simulink model "crazyflie_simulation_paper"  (R2019a)
settings: Solver=FixedStepAuto  StartTime=0.0  StopTime=50  FixedStep=Ts  RelTol=1e-3
values from neighbouring files (symbols this model uses):
  b = 0.033    [CHANGE_set_params_paper.m]    (also in set_params.m; set_params_paper.m)
  D_0 = 4/(Ts^2) + 4*zeta*omega_n/Ts + omega_n^2    (= 1011376)    [CHANGE_set_params_paper.m]    (also in set_params.m = 1057500; set_params_paper.m = 1057500)
  D_1 = -8/(Ts^2) + 2*omega_n^2    (= -1999872)    [CHANGE_set_params_paper.m]    (also in set_params.m = -1995000; set_params_paper.m = -1995000)
  D_2 = 4/(Ts^2) - 4*zeta*omega_n/Ts + omega_n^2    (= 988752)    [CHANGE_set_params_paper.m]    (also in set_params.m = 947500; set_params_paper.m = 947500)
  g = 9.81    [CHANGE_set_params_paper.m]    (also in set_params.m; set_params_paper.m)
  I_CF_1 = [16.823890  -1.224320  -0.716891 ... (first row only)    [CHANGE_set_params_paper.m]    (also in set_params.m; set_params_paper.m)
  I_CF_1_inv = inv(I_CF_1)    [CHANGE_set_params_paper.m]    (also in set_params.m; set_params_paper.m)
  I_rzz = 9.3e-9    (= 9.3e-09)    [CHANGE_set_params_paper.m]    (also in set_params.m; set_params_paper.m)
  k_f = 1.6e-4    (= 0.00016)    [CHANGE_set_params_paper.m]    (also in set_params.m; set_params_paper.m)
  k_m = 1e-6    (= 1e-06)    [CHANGE_set_params_paper.m]    (also in set_params.m; set_params_paper.m)
  kx = 10.25e-4    (= 0.001025)    [CHANGE_set_params_paper.m]    (also in set_params.m; set_params_paper.m)
  ky = 10.25e-4    (= 0.001025)    [CHANGE_set_params_paper.m]    (also in set_params.m; set_params_paper.m)
  kz = 7.553e-4    (= 0.0007553)    [CHANGE_set_params_paper.m]    (also in set_params.m; set_params_paper.m)
  l = 0.033    [CHANGE_set_params_paper.m]    (also in set_params.m; set_params_paper.m)
  m_CF = 0.028    [CHANGE_set_params_paper.m]    (also in set_params.m; set_params_paper.m)
  N_0 = omega_n^2    (= 64)    [CHANGE_set_params_paper.m]    (also in set_params.m = 2500; set_params_paper.m = 2500)
  N_1 = 2*omega_n^2    (= 128)    [CHANGE_set_params_paper.m]    (also in set_params.m = 5000; set_params_paper.m = 5000)
  N_2 = omega_n^2    (= 64)    [CHANGE_set_params_paper.m]    (also in set_params.m = 2500; set_params_paper.m = 2500)
  omegaR_init = [1; 1; 1; 1]*200    [CHANGE_set_params_paper.m]    (also in set_params.m; set_params_paper.m)
  T = 0.061658    [CHANGE_set_params_paper.m]    (also in inner_pd.m = 0.0666666666667; outer_pd_cs.m = 0.0666666666667; set_params.m = 0.0617; set_params_paper.m)
  T_init = m_CF*0.1    (= 0.0028)    [CHANGE_set_params_paper.m]    (also in set_params.m; set_params_paper.m)
  Ts = 1/500    (= 0.002)    [CHANGE_set_params_paper.m]    (also in inner_pd.m = 0.01; outer_pd_cs.m = 0.01; set_params.m; set_params_paper.m)
undefined symbols (not defined in the file or in its folder): DiscIntNeverNeededParam, sigbuilder_block
libraries: sharedutil x4, simulink x2
(part 1 of 2)
settings Model: Creator=evgheniivolodscoi  LastModifiedBy=evgheniivolodscoi

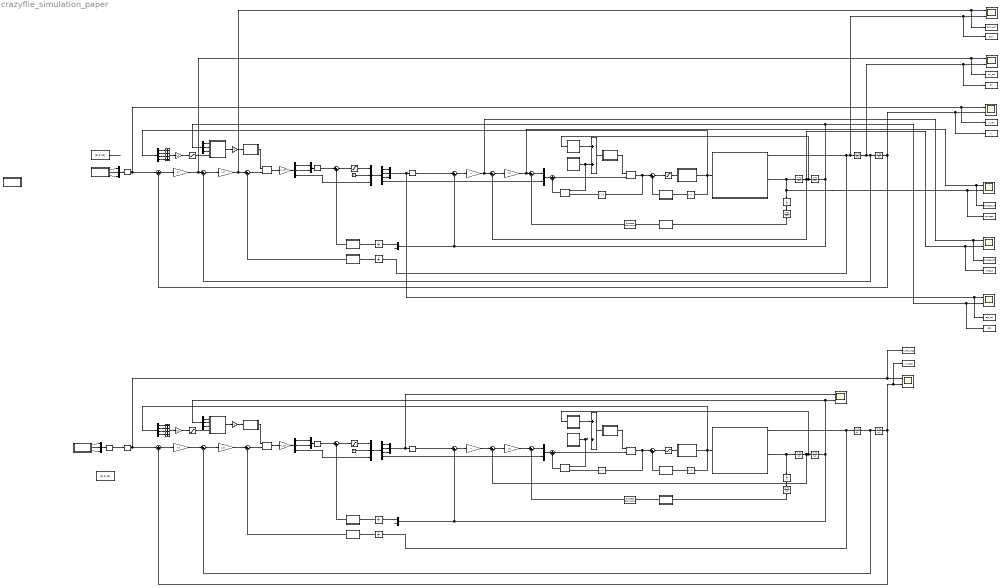
== system crazyflie_simulation_paper ==
  note: Outer Loop INDI
  note: Outer Loop INDI
  note: Inner Loop INDI
  note: Inner Loop INDI
  note: Outer Loop INDI
  note: Outer Loop INDI
  2nd order discrete Filter H(z) : Subsystem
  2nd order discrete Filter H(z)1 : Subsystem
  2nd order discrete Filter H(z)_1 : Subsystem
  2nd order discrete Filter H(z)_2 : Subsystem
  2nd order discrete Filter H(z)_3 : Subsystem
  2nd order discrete Filter H(z)_4 : Subsystem
  2nd order discrete Filter H(z)_5 : Subsystem
  2nd order discrete Filter H(z)_6 : Subsystem
  "Actuator Dynamics PT1_ " : Subsystem
  Actuator Dynamics PT1_ 1 : Subsystem
  Add : Sum
  Add1 : Sum  Inputs=++++
  Add2 : Sum
  Add3 : Sum  Inputs=++++
  Crazyflie Quadrotor Dynamics : Subsystem
  Crazyflie Quadrotor Dynamics1 : Subsystem
  Delay{,1..3} (4 alike) : Delay  DelayLength=1  InitialCondition=0
  Demux{,3,5,8} (4 alike) : Demux  Outputs=3
  Demux1 : Demux  Outputs=2
  Demux{2,4,7,9} (4 alike) : Demux
  Demux6 : Demux  Outputs=2
  Discrete Derivative : simulink/Discrete/Discrete Derivative  gainval=1.0  ICPrevScaledInput=0.0  OutMin=[]  OutMax=[]  OutDataType=fixdt(1, 16)  OutScaling=2^-10  DoSatur=off
  Discrete Derivative1 : simulink/Discrete/Discrete Derivative  gainval=1.0  ICPrevScaledInput=0.0  OutMin=[]  OutMax=[]  OutDataType=fixdt(1, 16)  OutScaling=2^-10  DoSatur=off
  Discrete-Time Integrator{,1..9} (10 alike) : DiscreteIntegrator  SampleTime=-1  ICPrevOutput=DiscIntNeverNeededParam  ICPrevScaledInput=DiscIntNeverNeededParam
  G : Subsystem
  G1 : Subsystem
  G2 : Subsystem
  G3 : Subsystem
  G4 : Subsystem
  G5 : Subsystem
  Gain : Gain  Gain=10
  Gain1 : Gain  Gain=4
  Gain10 : Gain  Gain=0.7
  Gain11 : Gain  Gain=1.8
  Gain12 : Gain  Gain=k_f
  Gain13 : Gain  Gain=-1
  Gain2 : Gain  Gain=m_CF
  Gain3 : Gain  Gain=0.7
  Gain4 : Gain  Gain=1.8
  Gain5 : Gain  Gain=k_f
  Gain6 : Gain  Gain=-1
  Gain7 : Gain  Gain=10
  Gain8 : Gain  Gain=4
  Gain9 : Gain  Gain=m_CF
  Matrix Multiply{,1..5} (6 alike) : Product  Multiplication=Matrix(*)
  Mux{,2,4,6} (4 alike) : Mux  Inputs=2
  Mux{1,3,5,7..9} (6 alike) : Mux  Inputs=3
  Pseudoinverse of u : MATLAB Function  TreatAsAtomicUnit=on
  "Pseudoinverse of u " : MATLAB Function  TreatAsAtomicUnit=on
  Pseudoinverse of u 1 : MATLAB Function  TreatAsAtomicUnit=on
  Pseudoinverse of u1 : MATLAB Function  TreatAsAtomicUnit=on
  Reshape{,1..6} (7 alike) : Reshape  OutputDimensionality=Column vector (2-D)
  Saturation : Saturate  UpperLimit=1000  LowerLimit=0
  Saturation1 : Saturate  UpperLimit=60/180*pi  LowerLimit=-60/180*pi
  Saturation2 : Saturate  UpperLimit=inf  LowerLimit=T_init
  Saturation3 : Saturate  UpperLimit=1000  LowerLimit=0
  Saturation4 : Saturate  UpperLimit=60/180*pi  LowerLimit=-60/180*pi
  Saturation5 : Saturate  UpperLimit=inf  LowerLimit=T_init
  Signal Builder1 : Subsystem  Tag=STV Subsys  LoadFcn=sigbuilder_block('load');  StartFcn=sigbuilder_block('start');  StopFcn=sigbuilder_block('stop');  ClipboardFcn=sigbuilder_block('clipboard');  mask(Sigbuilder block){tuvar=[0:10]}
      mask help: Simulink:masks:SigbuilderBlock_MD
      mask init:
      | if ~strcmp(get_param(bdroot(gcbh),'SimulationStatus'),'stopped') tuvar = sigbuilder_block('maskInit'); end
      settings: CopyFcn=sigbuilder_block('copy');  DeleteFcn=sigbuilder_block('delete');  ModelCloseFcn=sigbuilder_block('modelClose');  PreSaveFcn=sigbuilder_block('preSave');  PauseFcn=sigbuilder_block('pause');  ContinueFcn=sigbuilder_block('continue');  NameChangeFcn=sigbuilder_block('namechange');  OpenFcn=sigbuilder_block('open',[0 48.75 1440 596.25 ]);  CloseFcn=sigbuilder_block('close');
      mask Display: plot(0, 0, 100, 100,[2, 2, 32, 32, 2], [68, 8, 8, 68, 68],[32, 2], [38, 38], [32, 19, 2],[53, 60, 44], [32, 17, 17, 2],[16, 16, 31, 31]);txt = getActiveGroup(gcbh);text(2, 100, txt,'verticalAlignment', 'top');
  Signal Builder2 : Subsystem  Tag=STV Subsys  LoadFcn=sigbuilder_block('load');  StartFcn=sigbuilder_block('start');  StopFcn=sigbuilder_block('stop');  ClipboardFcn=sigbuilder_block('clipboard');  mask(Sigbuilder block){tuvar=[0:10]}
      mask help: Simulink:masks:SigbuilderBlock_MD
      mask init:
      | if ~strcmp(get_param(bdroot(gcbh),'SimulationStatus'),'stopped') tuvar = sigbuilder_block('maskInit'); end
      settings: CopyFcn=sigbuilder_block('copy');  DeleteFcn=sigbuilder_block('delete');  ModelCloseFcn=sigbuilder_block('modelClose');  PreSaveFcn=sigbuilder_block('preSave');  PauseFcn=sigbuilder_block('pause');  ContinueFcn=sigbuilder_block('continue');  NameChangeFcn=sigbuilder_block('namechange');  OpenFcn=sigbuilder_block('open',[0 48.75 1440 555 ]);  CloseFcn=sigbuilder_block('close');
      mask Display: plot(0, 0, 100, 100,[2, 2, 32, 32, 2], [68, 8, 8, 68, 68],[32, 2], [38, 38], [32, 19, 2],[53, 60, 44], [32, 17, 17, 2],[16, 16, 31, 31]);txt = getActiveGroup(gcbh);text(2, 100, txt,'verticalAlignment', 'top');
  Signal Builder3 : Subsystem  Tag=STV Subsys  LoadFcn=sigbuilder_block('load');  StartFcn=sigbuilder_block('start');  StopFcn=sigbuilder_block('stop');  ClipboardFcn=sigbuilder_block('clipboard');  mask(Sigbuilder block){tuvar=[0:10]}
      mask help: Simulink:masks:SigbuilderBlock_MD
      mask init:
      | if ~strcmp(get_param(bdroot(gcbh),'SimulationStatus'),'stopped') tuvar = sigbuilder_block('maskInit'); end
      settings: CopyFcn=sigbuilder_block('copy');  DeleteFcn=sigbuilder_block('delete');  ModelCloseFcn=sigbuilder_block('modelClose');  PreSaveFcn=sigbuilder_block('preSave');  PauseFcn=sigbuilder_block('pause');  ContinueFcn=sigbuilder_block('continue');  NameChangeFcn=sigbuilder_block('namechange');  OpenFcn=sigbuilder_block('open',[0 48.75 1440 596.25 ]);  CloseFcn=sigbuilder_block('close');
      mask Display: plot(0, 0, 100, 100,[2, 2, 32, 32, 2], [68, 8, 8, 68, 68],[32, 2], [38, 38], [32, 19, 2],[53, 60, 44], [32, 17, 17, 2],[16, 16, 31, 31]);txt = getActiveGroup(gcbh);text(2, 100, txt,'verticalAlignment', 'top');
  Sum{,1,8..10,17} (6 alike) : Sum  Inputs=|++
  Sum{2..7,11..16} (12 alike) : Sum  Inputs=|+-
  To Workspace : ToWorkspace  VariableName=xi  SampleTime=-1
  To Workspace1 : ToWorkspace  VariableName=xi_ref  SampleTime=-1
  To Workspace10 : ToWorkspace  VariableName=dxi  SampleTime=-1
  To Workspace11 : ToWorkspace  VariableName=dxi_ref  SampleTime=-1
  To Workspace12 : ToWorkspace  VariableName=domega  SampleTime=-1
  To Workspace13 : ToWorkspace  VariableName=domega_ref  SampleTime=-1
  To Workspace2 : ToWorkspace  VariableName=xi_nog2  SampleTime=-1
  To Workspace3 : ToWorkspace  VariableName=xi_ref_nog2  SampleTime=-1
  To Workspace4 : ToWorkspace  VariableName=eta  SampleTime=-1
  To Workspace5 : ToWorkspace  VariableName=eta_ref  SampleTime=-1
  To Workspace6 : ToWorkspace  VariableName=omega  SampleTime=-1
  To Workspace7 : ToWorkspace  VariableName=omega_ref  SampleTime=-1
  To Workspace8 : ToWorkspace  VariableName=ddxi  SampleTime=-1
  To Workspace9 : ToWorkspace  VariableName=ddxi_ref  SampleTime=-1
  Unit Delay{,1..5} (6 alike) : UnitDelay  SampleTime=-1  HasFrameUpgradeWarning=on
  const1 : Constant  Value=[6; 5; 10]
  const3 : Constant  Value=[6; 5; 10]
  "ddxi " : Scope  NumInputPorts=2
  domega_ref domega : Scope  NumInputPorts=2
  "dxi " : Scope  NumInputPorts=2
  eta_ref eta : Scope  NumInputPorts=2
  eta_ref eta1 : Scope  NumInputPorts=2
  omega_ref omega : Scope  NumInputPorts=2
  psi_c : Constant  Value=0
  psi_c1 : Constant  Value=0
  xi : Scope  NumInputPorts=2
  xi1 : Scope  NumInputPorts=2
  wires:
  G1/1(G1) -> Add/1
  G2/1(G2) -> Add/2, Matrix Multiply/1
  Matrix Multiply1/1 -> Sum1/1, Delay/1  "omegaR_tilde"
  Delay/1 -> Matrix Multiply/2
  Matrix Multiply/1 -> Sum/2
  Sum/1 -> Matrix Multiply1/2
  Mux/1 -> Sum/1
  Sum1/1 -> Saturation/1  "omegaR_c"
  2nd order discrete Filter H(z)/1(Y_z) -> Sum1/2  "omegaR_f"
  Delay1/1 -> 2nd order discrete Filter H(z)/1(U_z)  "omegaR_0"
  "Actuator Dynamics PT1_ "/1(y) -> Demux4/1, Delay1/1, Crazyflie Quadrotor Dynamics/1(omegaR)  "omegaR"
  Add/1 -> Pseudoinverse of u/1(u)
  Sum2/1 -> Mux/1  "d_p_err d_q_err d_r_err"
  Discrete Derivative/1 -> Sum2/2  "d_p_f d_q_f d_r_f"
  Gain/1 -> To Workspace13/1, domega_ref domega/1, Sum2/1  "dp_ref dq_ref dr_ref"
  Sum3/1 -> Gain/1  "p_err q_err r_err"
  Gain1/1 -> To Workspace7/1, omega_ref omega/1, Sum3/1  "p_ref q_ref r_ref"
  Discrete-Time Integrator1/1 -> To Workspace6/1, omega_ref omega/2, Sum3/2, G1/1(p q r), Discrete-Time Integrator2/1  "p q r"
  Sum4/1 -> Gain1/1  "phi_err theta_err psi_err"
  Discrete-Time Integrator/1 -> 2nd order discrete Filter H(z)_2/1(U_z)  "p_0 q_0 r_0"
  2nd order discrete Filter H(z)_2/1(Y_z) -> Discrete Derivative/1  "p_f q_f r_f"
  Crazyflie Quadrotor Dynamics/4(d_pqr) -> To Workspace12/1, domega_ref domega/2, Unit Delay/1, Discrete-Time Integrator1/1  "d_p d_q d_r"
  Unit Delay/1 -> Discrete-Time Integrator/1
  Gain2/1 -> Demux/1
  Sum5/1 -> Matrix Multiply2/2  "dd_xi_err"
  Gain4/1 -> To Workspace9/1, "ddxi "/1, Sum5/1  "dd_xi_ref"
  Gain3/1 -> To Workspace11/1, "dxi "/1, Sum6/1  "d_xi_ref"
  Sum7/1 -> Gain3/1  "xi_err"
  Discrete-Time Integrator4/1 -> To Workspace/1, xi/2, Sum7/2  "xi"
  Reshape2/1 -> Sum7/1, To Workspace1/1, xi/1  "xi_ref"
  Matrix Multiply2/1 -> Gain2/1
  Reshape1/1 -> Sum8/1  "phi_tilde theta_tilde"
  2nd order discrete Filter H(z)_3/1(Y_z) -> Sum8/2  "phi_f theta_f"
  Sum8/1 -> Saturation1/1  "phi_c theta_c"
  Unit Delay1/1 -> 2nd order discrete Filter H(z)_3/1(U_z)  "phi_0 theta_0"
  Demux1/1 -> Unit Delay1/1  "phi theta"
  Demux1/2 -> ?  "psi"
  Crazyflie Quadrotor Dynamics/1(d_V_O) -> To Workspace8/1, "ddxi "/2, Discrete-Time Integrator3/1, Unit Delay2/1  "dd_xi"
  Discrete-Time Integrator2/1 -> Demux3/1, To Workspace4/1, eta_ref eta/2, Demux1/1, Sum4/2  "phi theta psi"
  Mux1/1 -> To Workspace5/1, eta_ref eta/1, Reshape/1  "phi_ref theta_ref psi_ref"
  Demux2/2 -> Mux1/2
  Demux2/1 -> Mux1/1
  Demux2/3 -> Mux1/3
  Demux2/4 -> Mux/2  "T_tilde"
  Reshape/1 -> Sum4/1  "phi_ref theta_ref psi_ref"
  Pseudoinverse of u/1(y) -> Matrix Multiply1/1
  Demux/1 -> Mux2/1  "phi_tilde"
  Demux/2 -> Mux2/2  "theta_tilde"
  Demux/3 -> Mux3/3  "T_tilde"
  Mux2/1 -> Reshape1/1
  psi_c/1 -> Mux3/2
  Mux3/1 -> Demux2/1
  "Pseudoinverse of u "/1(y) -> Matrix Multiply2/1
  Demux3/1 -> G/1(phi)
  Demux3/2 -> G/2(theta)
  Demux3/3 -> G/3(psi)
  Demux4/1 -> Add1/1
  Demux4/2 -> Add1/2
  Demux4/3 -> Add1/3
  Demux4/4 -> Add1/4
  Add1/1 -> Gain5/1
  Gain5/1 -> Saturation2/1
  2nd order discrete Filter H(z)_4/1(Y_z) -> Sum5/2  "dd_xi_f"
  Unit Delay2/1 -> 2nd order discrete Filter H(z)_4/1(U_z)  "dd_xi_0"
  Discrete-Time Integrator3/1 -> To Workspace10/1, "dxi "/2, Sum6/2, Discrete-Time Integrator4/1  "d_xi_f"
  Sum6/1 -> Gain4/1  "d_xi_err"
  G/1(G) -> Gain6/1
  Saturation/1 -> "Actuator Dynamics PT1_ "/1(u)
  Saturation1/1 -> Mux3/1
  Saturation2/1 -> G/4(T)
  Gain6/1 -> "Pseudoinverse of u "/1(u)
  const1/1 -> ?  "xi_ref"
  psi_c1/1 -> Mux7/2
  Delay3/1 -> 2nd order discrete Filter H(z)1/1(U_z)  "omegaR_0"
  Crazyflie Quadrotor Dynamics1/4(d_pqr) -> Discrete-Time Integrator6/1, Unit Delay3/1  "d_p d_q d_r"
  Reshape3/1 -> Sum13/1  "phi_ref theta_ref psi_ref"
  Demux5/1 -> Mux6/1  "phi_tilde"
  Mux6/1 -> Reshape4/1
  Pseudoinverse of u1/1(y) -> Matrix Multiply4/1
  Mux4/1 -> Sum9/1
  Delay2/1 -> Matrix Multiply3/2
  Demux9/3 -> Add3/3
  Sum10/1 -> Saturation3/1  "omegaR_c"
  Demux7/1 -> Mux5/1
  Demux6/1 -> Unit Delay4/1  "phi theta"
  2nd order discrete Filter H(z)_1/1(Y_z) -> Discrete Derivative1/1  "p_f q_f r_f"
  Sum15/1 -> Gain11/1  "d_xi_err"
  G3/1(G) -> Gain13/1
  Gain8/1 -> Sum12/1  "p_ref q_ref r_ref"
  Discrete-Time Integrator8/1 -> Sum15/2, Discrete-Time Integrator9/1  "d_xi_f"
  Demux9/2 -> Add3/2
  Demux7/3 -> Mux5/3
  Demux7/2 -> Mux5/2
  Gain12/1 -> Saturation5/1
  Discrete Derivative1/1 -> Sum11/2  "d_p_f d_q_f d_r_f"
  Sum12/1 -> Gain7/1  "p_err q_err r_err"
  Sum11/1 -> Mux4/1  "d_p_err d_q_err d_r_err"
  Unit Delay4/1 -> 2nd order discrete Filter H(z)_5/1(U_z)  "phi_0 theta_0"
  Mux5/1 -> eta_ref eta1/1, Reshape3/1  "phi_ref theta_ref psi_ref"
  Sum14/1 -> Matrix Multiply5/2  "dd_xi_err"
  Pseudoinverse of u 1/1(y) -> Matrix Multiply5/1
  Discrete-Time Integrator9/1 -> To Workspace2/1, xi1/2, Sum16/2  "xi"
  Matrix Multiply5/1 -> Gain9/1
  Add3/1 -> Gain12/1
  Actuator Dynamics PT1_ 1/1(y) -> Demux9/1, Delay3/1, Crazyflie Quadrotor Dynamics1/1(omegaR)  "omegaR"
  Gain9/1 -> Demux5/1
  Demux8/3 -> G3/3(psi)
  Demux9/1 -> Add3/1
  Matrix Multiply4/1 -> Sum10/1, Delay2/1  "omegaR_tilde"
  Demux8/1 -> G3/1(phi)
  Saturation4/1 -> Mux7/1
  Demux6/2 -> ?  "psi"
  Gain13/1 -> Pseudoinverse of u 1/1(u)
  Reshape5/1 -> Sum16/1, To Workspace3/1, xi1/1  "xi_ref"
  Unit Delay3/1 -> Discrete-Time Integrator5/1
  Gain11/1 -> Sum14/1  "dd_xi_ref"
  Sum9/1 -> Matrix Multiply4/2
  Discrete-Time Integrator5/1 -> 2nd order discrete Filter H(z)_1/1(U_z)  "p_0 q_0 r_0"
  G4/1(G1) -> Add2/1
  G5/1(G2) -> Matrix Multiply3/1
  Add2/1 -> Pseudoinverse of u1/1(u)
  Gain7/1 -> Sum11/1  "dp_ref dq_ref dr_ref"
  Demux5/2 -> Mux6/2  "theta_tilde"
  Sum13/1 -> Gain8/1  "phi_err theta_err psi_err"
  Demux5/3 -> Mux7/3  "T_tilde"
  2nd order discrete Filter H(z)_5/1(Y_z) -> Sum17/2  "phi_f theta_f"
  Reshape4/1 -> Sum17/1  "phi_tilde theta_tilde"
  Crazyflie Quadrotor Dynamics1/1(d_V_O) -> Unit Delay5/1, Discrete-Time Integrator8/1  "dd_xi"
  Matrix Multiply3/1 -> Sum9/2
  Sum17/1 -> Saturation4/1  "phi_c theta_c"
  2nd order discrete Filter H(z)_6/1(Y_z) -> Sum14/2  "dd_xi_f"
  Gain10/1 -> Sum15/1  "d_xi_ref"
  Demux9/4 -> Add3/4
  Sum16/1 -> Gain10/1  "xi_err"
  Discrete-Time Integrator7/1 -> eta_ref eta1/2, Demux8/1, Demux6/1, Sum13/2  "phi theta psi"
  Demux7/4 -> Mux4/2  "T_tilde"
  Saturation5/1 -> G3/4(T)
  Unit Delay5/1 -> 2nd order discrete Filter H(z)_6/1(U_z)  "dd_xi_0"
  Saturation3/1 -> Actuator Dynamics PT1_ 1/1(u)
  Discrete-Time Integrator6/1 -> Sum12/2, G4/1(p q r), Discrete-Time Integrator7/1  "p q r"
  Mux7/1 -> Demux7/1
  2nd order discrete Filter H(z)1/1(Y_z) -> Sum10/2  "omegaR_f"
  Demux8/2 -> G3/2(theta)
  Mux8/1 -> Reshape2/1
  Signal Builder1/1(Signal 1) -> Mux8/1
  Signal Builder1/2(Signal 2) -> Mux8/2
  Signal Builder1/3(Signal 3) -> Mux8/3
  Signal Builder3/3(Signal 3) -> Mux9/3
  Signal Builder3/2(Signal 2) -> Mux9/2
  Signal Builder3/1(Signal 1) -> Mux9/1
  Mux9/1 -> Reshape6/1
  Reshape6/1 -> Reshape5/1  "xi_ref"

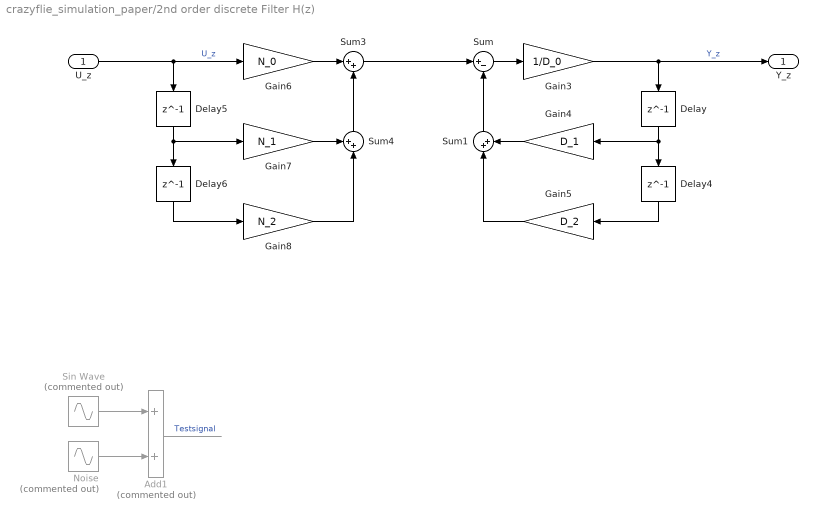
== system crazyflie_simulation_paper/2nd order discrete Filter H(z) ==
  U_z : Inport
  Add1 : Sum  Commented=on
  Delay{,4..6} (4 alike) : Delay  DelayLength=1  InitialCondition=0
  Gain3 : Gain  Gain=1/D_0
  Gain4 : Gain  Gain=D_1
  Gain5 : Gain  Gain=D_2
  Gain6 : Gain  Gain=N_0
  Gain7 : Gain  Gain=N_1
  Gain8 : Gain  Gain=N_2
  Noise : Sin  Commented=on  Amplitude=0.15  Frequency=10*2*pi  SampleTime=0
  Sin Wave : Sin  Commented=on  Frequency=100/2/pi*2*pi  SampleTime=0
  Sum : Sum  Inputs=|+-
  Sum1 : Sum  Inputs=|++
  Sum3 : Sum  Inputs=|++
  Sum4 : Sum  Inputs=++|
  Y_z : Outport
  wires:
  Add1/1 -> ?  "Testsignal"
  Sin Wave/1 -> Add1/1
  Noise/1 -> Add1/2
  Delay6/1 -> Gain8/1
  Gain8/1 -> Sum4/2
  Sum4/1 -> Sum3/2
  Gain7/1 -> Sum4/1
  Delay5/1 -> Gain7/1, Delay6/1
  U_z/1 -> Gain6/1, Delay5/1  "U_z"
  Gain6/1 -> Sum3/1
  Sum3/1 -> Sum/1
  Gain5/1 -> Sum1/1
  Gain4/1 -> Sum1/2
  Gain3/1 -> Delay/1, Y_z/1  "Y_z"
  Sum1/1 -> Sum/2
  Delay4/1 -> Gain5/1
  Delay/1 -> Gain4/1, Delay4/1
  Sum/1 -> Gain3/1

== system crazyflie_simulation_paper/2nd order discrete Filter H(z)1 ==
  U_z : Inport
  Add1 : Sum  Commented=on
  Delay{,4..6} (4 alike) : Delay  DelayLength=1  InitialCondition=0
  Gain3 : Gain  Gain=1/D_0
  Gain4 : Gain  Gain=D_1
  Gain5 : Gain  Gain=D_2
  Gain6 : Gain  Gain=N_0
  Gain7 : Gain  Gain=N_1
  Gain8 : Gain  Gain=N_2
  Noise : Sin  Commented=on  Amplitude=0.15  Frequency=10*2*pi  SampleTime=0
  Sin Wave : Sin  Commented=on  Frequency=100/2/pi*2*pi  SampleTime=0
  Sum : Sum  Inputs=|+-
  Sum1 : Sum  Inputs=|++
  Sum3 : Sum  Inputs=|++
  Sum4 : Sum  Inputs=++|
  Y_z : Outport
  wires:
  Add1/1 -> ?  "Testsignal"
  Sin Wave/1 -> Add1/1
  Noise/1 -> Add1/2
  Delay6/1 -> Gain8/1
  Gain8/1 -> Sum4/2
  Sum4/1 -> Sum3/2
  Gain7/1 -> Sum4/1
  Delay5/1 -> Gain7/1, Delay6/1
  U_z/1 -> Gain6/1, Delay5/1  "U_z"
  Gain6/1 -> Sum3/1
  Sum3/1 -> Sum/1
  Gain5/1 -> Sum1/1
  Gain4/1 -> Sum1/2
  Gain3/1 -> Delay/1, Y_z/1  "Y_z"
  Sum1/1 -> Sum/2
  Delay4/1 -> Gain5/1
  Delay/1 -> Gain4/1, Delay4/1
  Sum/1 -> Gain3/1

== system crazyflie_simulation_paper/2nd order discrete Filter H(z)_1 ==
  U_z : Inport
  Add1 : Sum  Commented=on
  Delay{,4..6} (4 alike) : Delay  DelayLength=1  InitialCondition=0
  Gain3 : Gain  Gain=1/D_0
  Gain4 : Gain  Gain=D_1
  Gain5 : Gain  Gain=D_2
  Gain6 : Gain  Gain=N_0
  Gain7 : Gain  Gain=N_1
  Gain8 : Gain  Gain=N_2
  Noise : Sin  Commented=on  Amplitude=0.15  Frequency=10*2*pi  SampleTime=0
  Sin Wave : Sin  Commented=on  Frequency=100/2/pi*2*pi  SampleTime=0
  Sum : Sum  Inputs=|+-
  Sum1 : Sum  Inputs=|++
  Sum3 : Sum  Inputs=|++
  Sum4 : Sum  Inputs=++|
  Y_z : Outport
  wires:
  Sum/1 -> Gain3/1
  Delay/1 -> Delay4/1, Gain4/1
  Delay4/1 -> Gain5/1
  Sum1/1 -> Sum/2
  Gain3/1 -> Y_z/1, Delay/1  "Y_z"
  Gain4/1 -> Sum1/2
  Gain5/1 -> Sum1/1
  Sum3/1 -> Sum/1
  Gain6/1 -> Sum3/1
  U_z/1 -> Delay5/1, Gain6/1  "U_z"
  Delay5/1 -> Delay6/1, Gain7/1
  Gain7/1 -> Sum4/1
  Sum4/1 -> Sum3/2
  Gain8/1 -> Sum4/2
  Delay6/1 -> Gain8/1
  Noise/1 -> Add1/2
  Sin Wave/1 -> Add1/1
  Add1/1 -> ?  "Testsignal"

== system crazyflie_simulation_paper/2nd order discrete Filter H(z)_2 ==
  U_z : Inport
  Add1 : Sum  Commented=on
  Delay{,4..6} (4 alike) : Delay  DelayLength=1  InitialCondition=0
  Gain3 : Gain  Gain=1/D_0
  Gain4 : Gain  Gain=D_1
  Gain5 : Gain  Gain=D_2
  Gain6 : Gain  Gain=N_0
  Gain7 : Gain  Gain=N_1
  Gain8 : Gain  Gain=N_2
  Noise : Sin  Commented=on  Amplitude=0.15  Frequency=10*2*pi  SampleTime=0
  Sin Wave : Sin  Commented=on  Frequency=100/2/pi*2*pi  SampleTime=0
  Sum : Sum  Inputs=|+-
  Sum1 : Sum  Inputs=|++
  Sum3 : Sum  Inputs=|++
  Sum4 : Sum  Inputs=++|
  Y_z : Outport
  wires:
  Sum/1 -> Gain3/1
  Delay/1 -> Delay4/1, Gain4/1
  Delay4/1 -> Gain5/1
  Sum1/1 -> Sum/2
  Gain3/1 -> Y_z/1, Delay/1  "Y_z"
  Gain4/1 -> Sum1/2
  Gain5/1 -> Sum1/1
  Sum3/1 -> Sum/1
  Gain6/1 -> Sum3/1
  U_z/1 -> Delay5/1, Gain6/1  "U_z"
  Delay5/1 -> Delay6/1, Gain7/1
  Gain7/1 -> Sum4/1
  Sum4/1 -> Sum3/2
  Gain8/1 -> Sum4/2
  Delay6/1 -> Gain8/1
  Noise/1 -> Add1/2
  Sin Wave/1 -> Add1/1
  Add1/1 -> ?  "Testsignal"

== system crazyflie_simulation_paper/2nd order discrete Filter H(z)_3 ==
  U_z : Inport
  Add1 : Sum  Commented=on
  Delay{,4..6} (4 alike) : Delay  DelayLength=1  InitialCondition=0
  Gain3 : Gain  Gain=1/D_0
  Gain4 : Gain  Gain=D_1
  Gain5 : Gain  Gain=D_2
  Gain6 : Gain  Gain=N_0
  Gain7 : Gain  Gain=N_1
  Gain8 : Gain  Gain=N_2
  Noise : Sin  Commented=on  Amplitude=0.15  Frequency=10*2*pi  SampleTime=0
  Sin Wave : Sin  Commented=on  Frequency=100/2/pi*2*pi  SampleTime=0
  Sum : Sum  Inputs=|+-
  Sum1 : Sum  Inputs=|++
  Sum3 : Sum  Inputs=|++
  Sum4 : Sum  Inputs=++|
  Y_z : Outport
  wires:
  Add1/1 -> ?  "Testsignal"
  Sin Wave/1 -> Add1/1
  Noise/1 -> Add1/2
  Delay6/1 -> Gain8/1
  Gain8/1 -> Sum4/2
  Sum4/1 -> Sum3/2
  Gain7/1 -> Sum4/1
  Delay5/1 -> Gain7/1, Delay6/1
  U_z/1 -> Gain6/1, Delay5/1  "U_z"
  Gain6/1 -> Sum3/1
  Sum3/1 -> Sum/1
  Gain5/1 -> Sum1/1
  Gain4/1 -> Sum1/2
  Gain3/1 -> Delay/1, Y_z/1  "Y_z"
  Sum1/1 -> Sum/2
  Delay4/1 -> Gain5/1
  Delay/1 -> Gain4/1, Delay4/1
  Sum/1 -> Gain3/1

== system crazyflie_simulation_paper/2nd order discrete Filter H(z)_4 ==
  U_z : Inport
  Add1 : Sum  Commented=on
  Delay{,4..6} (4 alike) : Delay  DelayLength=1  InitialCondition=0
  Gain3 : Gain  Gain=1/D_0
  Gain4 : Gain  Gain=D_1
  Gain5 : Gain  Gain=D_2
  Gain6 : Gain  Gain=N_0
  Gain7 : Gain  Gain=N_1
  Gain8 : Gain  Gain=N_2
  Noise : Sin  Commented=on  Amplitude=0.15  Frequency=10*2*pi  SampleTime=0
  Sin Wave : Sin  Commented=on  Frequency=100/2/pi*2*pi  SampleTime=0
  Sum : Sum  Inputs=|+-
  Sum1 : Sum  Inputs=|++
  Sum3 : Sum  Inputs=|++
  Sum4 : Sum  Inputs=++|
  Y_z : Outport
  wires:
  Sum/1 -> Gain3/1
  Delay/1 -> Delay4/1, Gain4/1
  Delay4/1 -> Gain5/1
  Sum1/1 -> Sum/2
  Gain3/1 -> Y_z/1, Delay/1  "Y_z"
  Gain4/1 -> Sum1/2
  Gain5/1 -> Sum1/1
  Sum3/1 -> Sum/1
  Gain6/1 -> Sum3/1
  U_z/1 -> Delay5/1, Gain6/1  "U_z"
  Delay5/1 -> Delay6/1, Gain7/1
  Gain7/1 -> Sum4/1
  Sum4/1 -> Sum3/2
  Gain8/1 -> Sum4/2
  Delay6/1 -> Gain8/1
  Noise/1 -> Add1/2
  Sin Wave/1 -> Add1/1
  Add1/1 -> ?  "Testsignal"

== system crazyflie_simulation_paper/2nd order discrete Filter H(z)_5 ==
  U_z : Inport
  Add1 : Sum  Commented=on
  Delay{,4..6} (4 alike) : Delay  DelayLength=1  InitialCondition=0
  Gain3 : Gain  Gain=1/D_0
  Gain4 : Gain  Gain=D_1
  Gain5 : Gain  Gain=D_2
  Gain6 : Gain  Gain=N_0
  Gain7 : Gain  Gain=N_1
  Gain8 : Gain  Gain=N_2
  Noise : Sin  Commented=on  Amplitude=0.15  Frequency=10*2*pi  SampleTime=0
  Sin Wave : Sin  Commented=on  Frequency=100/2/pi*2*pi  SampleTime=0
  Sum : Sum  Inputs=|+-
  Sum1 : Sum  Inputs=|++
  Sum3 : Sum  Inputs=|++
  Sum4 : Sum  Inputs=++|
  Y_z : Outport
  wires:
  Add1/1 -> ?  "Testsignal"
  Sin Wave/1 -> Add1/1
  Noise/1 -> Add1/2
  Delay6/1 -> Gain8/1
  Gain8/1 -> Sum4/2
  Sum4/1 -> Sum3/2
  Gain7/1 -> Sum4/1
  Delay5/1 -> Gain7/1, Delay6/1
  U_z/1 -> Gain6/1, Delay5/1  "U_z"
  Gain6/1 -> Sum3/1
  Sum3/1 -> Sum/1
  Gain5/1 -> Sum1/1
  Gain4/1 -> Sum1/2
  Gain3/1 -> Delay/1, Y_z/1  "Y_z"
  Sum1/1 -> Sum/2
  Delay4/1 -> Gain5/1
  Delay/1 -> Gain4/1, Delay4/1
  Sum/1 -> Gain3/1

== system crazyflie_simulation_paper/2nd order discrete Filter H(z)_6 ==
  U_z : Inport
  Add1 : Sum  Commented=on
  Delay{,4..6} (4 alike) : Delay  DelayLength=1  InitialCondition=0
  Gain3 : Gain  Gain=1/D_0
  Gain4 : Gain  Gain=D_1
  Gain5 : Gain  Gain=D_2
  Gain6 : Gain  Gain=N_0
  Gain7 : Gain  Gain=N_1
  Gain8 : Gain  Gain=N_2
  Noise : Sin  Commented=on  Amplitude=0.15  Frequency=10*2*pi  SampleTime=0
  Sin Wave : Sin  Commented=on  Frequency=100/2/pi*2*pi  SampleTime=0
  Sum : Sum  Inputs=|+-
  Sum1 : Sum  Inputs=|++
  Sum3 : Sum  Inputs=|++
  Sum4 : Sum  Inputs=++|
  Y_z : Outport
  wires:
  Sum/1 -> Gain3/1
  Delay/1 -> Delay4/1, Gain4/1
  Delay4/1 -> Gain5/1
  Sum1/1 -> Sum/2
  Gain3/1 -> Y_z/1, Delay/1  "Y_z"
  Gain4/1 -> Sum1/2
  Gain5/1 -> Sum1/1
  Sum3/1 -> Sum/1
  Gain6/1 -> Sum3/1
  U_z/1 -> Delay5/1, Gain6/1  "U_z"
  Delay5/1 -> Delay6/1, Gain7/1
  Gain7/1 -> Sum4/1
  Sum4/1 -> Sum3/2
  Gain8/1 -> Sum4/2
  Delay6/1 -> Gain8/1
  Noise/1 -> Add1/2
  Sin Wave/1 -> Add1/1
  Add1/1 -> ?  "Testsignal"

== system crazyflie_simulation_paper/Actuator Dynamics PT1_  ==
  u : Inport
  Gain : Gain  Gain=1/T
  Integrator : Integrator  InitialCondition=omegaR_init
  Sum : Sum  Inputs=|+-
  y : Outport
  wires:
  Sum/1 -> Gain/1
  Gain/1 -> Integrator/1  "d_y"
  u/1 -> Sum/1
  Integrator/1 -> y/1, Sum/2  "y"

== system crazyflie_simulation_paper/Actuator Dynamics PT1_ 1 ==
  u : Inport
  Gain : Gain  Gain=1/T
  Integrator : Integrator  InitialCondition=omegaR_init
  Sum : Sum  Inputs=|+-
  y : Outport
  wires:
  Sum/1 -> Gain/1
  Gain/1 -> Integrator/1  "d_y"
  u/1 -> Sum/1
  Integrator/1 -> y/1, Sum/2  "y"

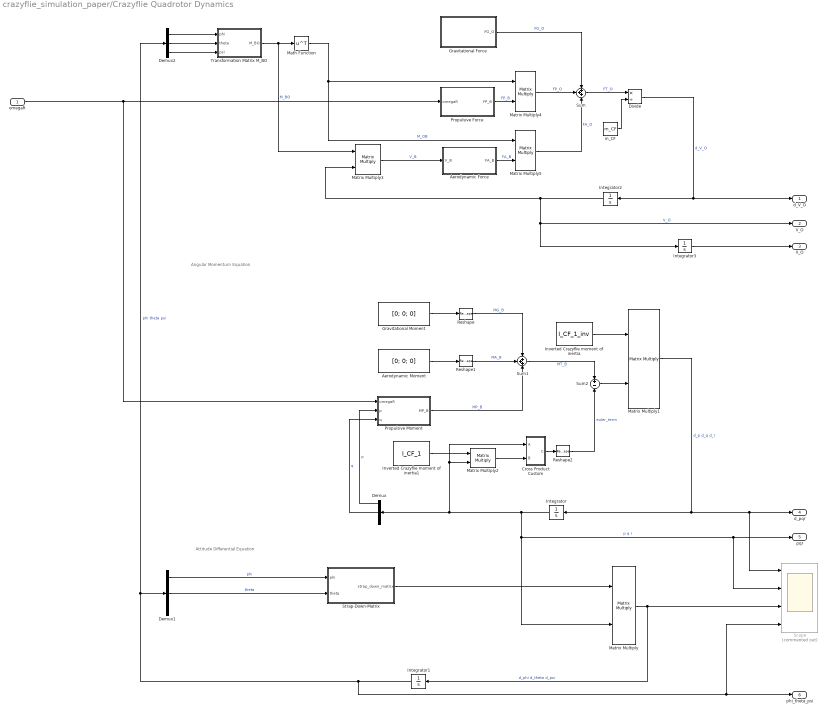
== system crazyflie_simulation_paper/Crazyflie Quadrotor Dynamics ==
  note: Attitude Differential Equation
  note: Angular Momentum Equation
  omegaR : Inport
  Aerodynamic Force : Subsystem
  Aerodynamic Moment : Constant  Value=[0; 0; 0]
  Cross Product Custom : Subsystem
  Demux : Demux  Outputs=3
  Demux1 : Demux  Outputs=3
  Demux2 : Demux  Outputs=3
  Divide : Product  Inputs=*/
  "Gravitational Force " : Subsystem
  Gravitational Moment : Constant  Value=[0; 0; 0]
  Integrator{,1..3} (4 alike) : Integrator  InitialCondition=[0; 0; 0]
  Inverted Crazyflie moment of inertia : Constant  Value=I_CF_1_inv
  Inverted Crazyflie moment of inertia1 : Constant  Value=I_CF_1
  Math Function : Math  Operator=transpose  SaturateOnIntegerOverflow=on
  Matrix Multiply{,1..5} (6 alike) : Product  Multiplication=Matrix(*)
  Propulsive Force : Subsystem
  Propulsive Moment : Subsystem
  Reshape : Reshape  OutputDimensionality=Column vector (2-D)
  Reshape1 : Reshape  OutputDimensionality=Column vector (2-D)
  Reshape2 : Reshape  OutputDimensionality=Column vector (2-D)
  Scope : Scope  Commented=on  NumInputPorts=4
  Strap-Down-Matrix : Subsystem
  Sum : Sum  Inputs=+++
  Sum1 : Sum  Inputs=+++
  Sum2 : Sum  Inputs=+-
  Transformation Matrix M_BO : Subsystem
  m_CF : Constant  Value=m_CF
  d_V_O : Outport
  V_O : Outport  Port=2
  X_O : Outport  Port=3
  d_pqr : Outport  Port=4
  pqr : Outport  Port=5
  phi_theta_psi : Outport  Port=6
  wires:
  Inverted Crazyflie moment of inertia1/1 -> Matrix Multiply2/1
  Sum2/1 -> Matrix Multiply1/2
  Integrator3/1 -> X_O/1
  Integrator2/1 -> Matrix Multiply3/2, V_O/1, Integrator3/1  "V_O"
  Divide/1 -> Integrator2/1, d_V_O/1  "d_V_O"
  omegaR/1 -> Propulsive Force/1(omegaR), Propulsive Moment/1(omegaR)
  Reshape2/1 -> Sum2/2  "euler_term"
  Reshape1/1 -> Sum1/2  "MA_B"
  Reshape/1 -> Sum1/1  "MG_B"
  Demux/2 -> Propulsive Moment/3(q)  "q"
  Sum1/1 -> Sum2/1  "MT_B"
  Demux1/1 -> Strap-Down-Matrix/1(phi)  "phi"
  Demux2/3 -> Transformation Matrix M_BO/3(psi)
  Strap-Down-Matrix/1(strap_down_matrix) -> Matrix Multiply/1
  Matrix Multiply5/1 -> Sum/3  "FA_O"
  Math Function/1 -> Matrix Multiply5/1, Matrix Multiply4/1  "M_OB"
  Demux2/1 -> Transformation Matrix M_BO/1(phi)
  Matrix Multiply3/1 -> Aerodynamic Force/1(V_B)  "V_B"
  Matrix Multiply/1 -> Scope/3, Integrator1/1  "d_phi d_theta d_psi"
  Cross Product Custom/1(C) -> Reshape2/1
  Matrix Multiply2/1 -> Cross Product Custom/2(B)
  Aerodynamic Force/1(FA_B) -> Matrix Multiply5/2  "FA_B"
  Transformation Matrix M_BO/1(M_BO) -> Math Function/1, Matrix Multiply3/1  "M_BO"
  Gravitational Moment/1 -> Reshape/1
  m_CF/1 -> Divide/2
  Demux2/2 -> Transformation Matrix M_BO/2(theta)
  Sum/1 -> Divide/1  "FT_O"
  Propulsive Moment/1(MP_B) -> Sum1/3  "MP_B"
  Matrix Multiply4/1 -> Sum/2  "FP_O"
  "Gravitational Force "/1(FG_O) -> Sum/1  "FG_O"
  Propulsive Force/1(FP_B) -> Matrix Multiply4/2  "FP_B"
  Integrator/1 -> pqr/1, Scope/2, Matrix Multiply/2, Matrix Multiply2/2, Cross Product Custom/1(A), Demux/1  "p q r"
  Demux/1 -> Propulsive Moment/2(p)  "p"
  Integrator1/1 -> phi_theta_psi/1, Scope/4, Demux1/1, Demux2/1  "phi theta psi"
  Inverted Crazyflie moment of inertia/1 -> Matrix Multiply1/1
  Demux1/2 -> Strap-Down-Matrix/2(theta)  "theta"
  Matrix Multiply1/1 -> d_pqr/1, Scope/1, Integrator/1  "d_p d_q d_r"
  Aerodynamic Moment/1 -> Reshape1/1

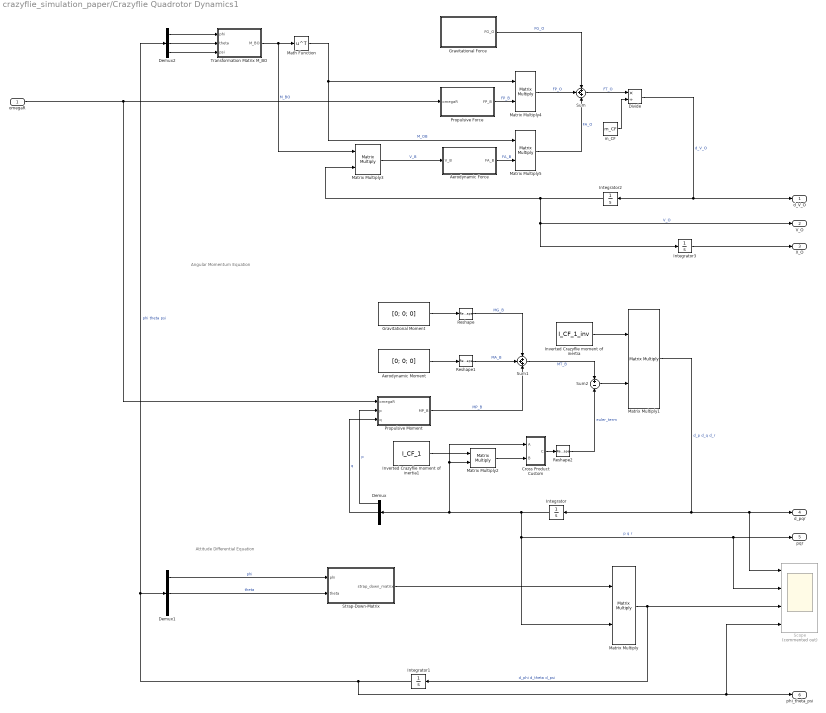
== system crazyflie_simulation_paper/Crazyflie Quadrotor Dynamics1 ==
  note: Attitude Differential Equation
  note: Angular Momentum Equation
  omegaR : Inport
  Aerodynamic Force : Subsystem
  Aerodynamic Moment : Constant  Value=[0; 0; 0]
  Cross Product Custom : Subsystem
  Demux : Demux  Outputs=3
  Demux1 : Demux  Outputs=3
  Demux2 : Demux  Outputs=3
  Divide : Product  Inputs=*/
  "Gravitational Force " : Subsystem
  Gravitational Moment : Constant  Value=[0; 0; 0]
  Integrator{,1..3} (4 alike) : Integrator  InitialCondition=[0; 0; 0]
  Inverted Crazyflie moment of inertia : Constant  Value=I_CF_1_inv
  Inverted Crazyflie moment of inertia1 : Constant  Value=I_CF_1
  Math Function : Math  Operator=transpose  SaturateOnIntegerOverflow=on
  Matrix Multiply{,1..5} (6 alike) : Product  Multiplication=Matrix(*)
  Propulsive Force : Subsystem
  Propulsive Moment : Subsystem
  Reshape : Reshape  OutputDimensionality=Column vector (2-D)
  Reshape1 : Reshape  OutputDimensionality=Column vector (2-D)
  Reshape2 : Reshape  OutputDimensionality=Column vector (2-D)
  Scope : Scope  Commented=on  NumInputPorts=4
  Strap-Down-Matrix : Subsystem
  Sum : Sum  Inputs=+++
  Sum1 : Sum  Inputs=+++
  Sum2 : Sum  Inputs=+-
  Transformation Matrix M_BO : Subsystem
  m_CF : Constant  Value=m_CF
  d_V_O : Outport
  V_O : Outport  Port=2
  X_O : Outport  Port=3
  d_pqr : Outport  Port=4
  pqr : Outport  Port=5
  phi_theta_psi : Outport  Port=6
  wires:
  Inverted Crazyflie moment of inertia1/1 -> Matrix Multiply2/1
  Sum2/1 -> Matrix Multiply1/2
  Integrator3/1 -> X_O/1
  Integrator2/1 -> Matrix Multiply3/2, V_O/1, Integrator3/1  "V_O"
  Divide/1 -> Integrator2/1, d_V_O/1  "d_V_O"
  omegaR/1 -> Propulsive Force/1(omegaR), Propulsive Moment/1(omegaR)
  Reshape2/1 -> Sum2/2  "euler_term"
  Reshape1/1 -> Sum1/2  "MA_B"
  Reshape/1 -> Sum1/1  "MG_B"
  Demux/2 -> Propulsive Moment/3(q)  "q"
  Sum1/1 -> Sum2/1  "MT_B"
  Demux1/1 -> Strap-Down-Matrix/1(phi)  "phi"
  Demux2/3 -> Transformation Matrix M_BO/3(psi)
  Strap-Down-Matrix/1(strap_down_matrix) -> Matrix Multiply/1
  Matrix Multiply5/1 -> Sum/3  "FA_O"
  Math Function/1 -> Matrix Multiply5/1, Matrix Multiply4/1  "M_OB"
  Demux2/1 -> Transformation Matrix M_BO/1(phi)
  Matrix Multiply3/1 -> Aerodynamic Force/1(V_B)  "V_B"
  Matrix Multiply/1 -> Scope/3, Integrator1/1  "d_phi d_theta d_psi"
  Cross Product Custom/1(C) -> Reshape2/1
  Matrix Multiply2/1 -> Cross Product Custom/2(B)
  Aerodynamic Force/1(FA_B) -> Matrix Multiply5/2  "FA_B"
  Transformation Matrix M_BO/1(M_BO) -> Math Function/1, Matrix Multiply3/1  "M_BO"
  Gravitational Moment/1 -> Reshape/1
  m_CF/1 -> Divide/2
  Demux2/2 -> Transformation Matrix M_BO/2(theta)
  Sum/1 -> Divide/1  "FT_O"
  Propulsive Moment/1(MP_B) -> Sum1/3  "MP_B"
  Matrix Multiply4/1 -> Sum/2  "FP_O"
  "Gravitational Force "/1(FG_O) -> Sum/1  "FG_O"
  Propulsive Force/1(FP_B) -> Matrix Multiply4/2  "FP_B"
  Integrator/1 -> pqr/1, Scope/2, Matrix Multiply/2, Matrix Multiply2/2, Cross Product Custom/1(A), Demux/1  "p q r"
  Demux/1 -> Propulsive Moment/2(p)  "p"
  Integrator1/1 -> phi_theta_psi/1, Scope/4, Demux1/1, Demux2/1  "phi theta psi"
  Inverted Crazyflie moment of inertia/1 -> Matrix Multiply1/1
  Demux1/2 -> Strap-Down-Matrix/2(theta)  "theta"
  Matrix Multiply1/1 -> d_pqr/1, Scope/1, Integrator/1  "d_p d_q d_r"
  Aerodynamic Moment/1 -> Reshape1/1

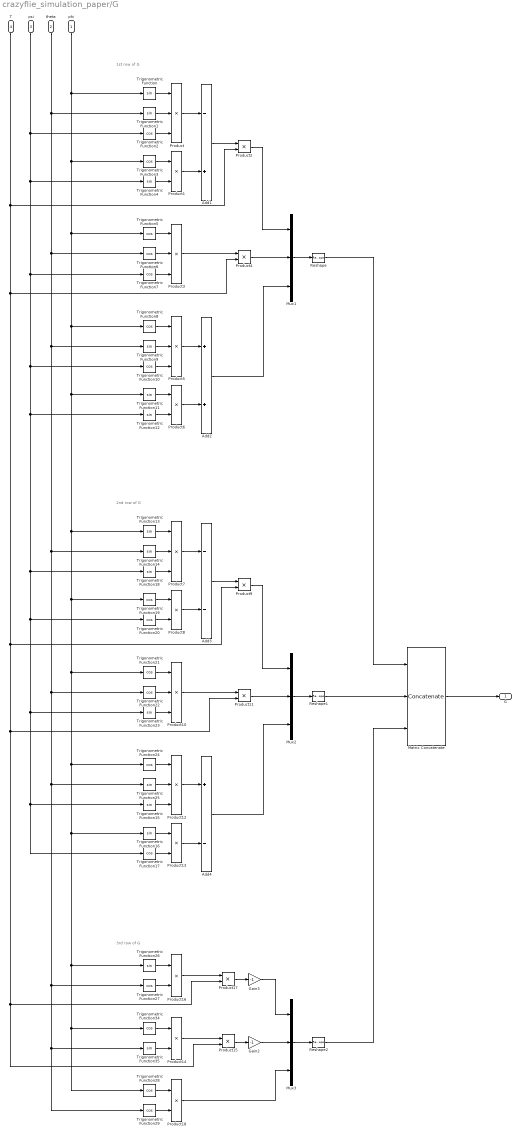
== system crazyflie_simulation_paper/G ==
  note: 1st row of G
  note: 2nd row of G
  note: 3rd row of G
  phi : Inport
  theta : Inport  Port=2
  psi : Inport  Port=3
  T : Inport  Port=4
  Add1 : Sum  Inputs=-+
  Add2 : Sum
  Add3 : Sum  Inputs=--
  Add4 : Sum  Inputs=+-
  Gain2 : Gain  Gain=-1
  Gain3 : Gain  Gain=-1
  Matrix Concatenate : Concatenate  NumInputs=3  Mode=Multidimensional array
  Mux1 : Mux  Inputs=3
  Mux2 : Mux  Inputs=3
  Mux3 : Mux  Inputs=3
  Product{,3,5,7,10,12} (6 alike) : Product  Inputs=3
  Product{1..2,4,6,8..9,11,13..18} (13 alike) : Product
  Reshape : Reshape  OutputDimensionality=Row vector (2-D)
  Reshape1 : Reshape  OutputDimensionality=Row vector (2-D)
  Reshape2 : Reshape  OutputDimensionality=Row vector (2-D)
  Trigonometric Function{,1,4,9,11..16,18,23,25..26,35} (15 alike) : Trigonometry
  Trigonometric Function{2..3,5..8,10,17,19..22,24,27..29,34} (17 alike) : Trigonometry  Operator=cos
  G : Outport
  wires:
  T/1 -> Product2/2, Product4/2, Product9/2, Product11/2, Product17/2, Product15/2
  Mux1/1 -> Reshape/1
  theta/1 -> Trigonometric Function1/1, Trigonometric Function6/1, Trigonometric Function9/1, Trigonometric Function14/1, Trigonometric Function22/1, Trigonometric Function25/1, Trigonometric Function27/1, Trigonometric Function35/1, Trigonometric Function29/1
  Trigonometric Function34/1 -> Product14/1
  Reshape/1 -> Matrix Concatenate/1
  psi/1 -> Trigonometric Function2/1, Trigonometric Function4/1, Trigonometric Function7/1, Trigonometric Function10/1, Trigonometric Function12/1, Trigonometric Function18/1, Trigonometric Function20/1, Trigonometric Function23/1, Trigonometric Function15/1, Trigonometric Function17/1
  Trigonometric Function25/1 -> Product12/2
  Trigonometric Function26/1 -> Product16/1
  Add1/1 -> Product2/1
  phi/1 -> Trigonometric Function3/1, Trigonometric Function8/1, Trigonometric Function13/1, Trigonometric Function19/1, Trigonometric Function21/1, Trigonometric Function24/1, Trigonometric Function26/1, Trigonometric Function34/1, Trigonometric Function28/1, Trigonometric Function16/1, Trigonometric Function11/1, Trigonometric Function5/1, Trigonometric Function/1
  Trigonometric Function15/1 -> Product12/3
  Trigonometric Function24/1 -> Product12/1
  Trigonometric Function20/1 -> Product8/2
  Product18/1 -> Mux3/3
  Product4/1 -> Mux1/2
  Mux3/1 -> Reshape2/1
  Product7/1 -> Add3/1
  Trigonometric Function6/1 -> Product3/2
  Matrix Concatenate/1 -> G/1
  Trigonometric Function7/1 -> Product3/3
  Trigonometric Function3/1 -> Product1/1
  Trigonometric Function29/1 -> Product18/2
  Trigonometric Function5/1 -> Product3/1
  Product1/1 -> Add1/2
  Trigonometric Function8/1 -> Product5/1
  Product6/1 -> Add2/2
  Product15/1 -> Gain2/1
  Mux2/1 -> Reshape1/1
  Product17/1 -> Gain3/1
  Gain2/1 -> Mux3/2
  Trigonometric Function17/1 -> Product13/2
  Product12/1 -> Add4/1
  Trigonometric Function19/1 -> Product8/1
  Product3/1 -> Product4/1
  Product9/1 -> Mux2/1
  Product16/1 -> Product17/1
  Add4/1 -> Mux2/3
  Trigonometric Function16/1 -> Product13/1
  Product8/1 -> Add3/2
  Trigonometric Function13/1 -> Product7/1
  Trigonometric Function28/1 -> Product18/1
  Gain3/1 -> Mux3/1
  Add3/1 -> Product9/1
  Trigonometric Function35/1 -> Product14/2
  Trigonometric Function18/1 -> Product7/3
  Product14/1 -> Product15/1
  Trigonometric Function/1 -> Product/1
  Product11/1 -> Mux2/2
  Product13/1 -> Add4/2
  Trigonometric Function21/1 -> Product10/1
  Product10/1 -> Product11/1
  Trigonometric Function22/1 -> Product10/2
  Trigonometric Function23/1 -> Product10/3
  Trigonometric Function14/1 -> Product7/2
  Reshape2/1 -> Matrix Concatenate/3
  Trigonometric Function1/1 -> Product/2
  Product2/1 -> Mux1/1
  Trigonometric Function11/1 -> Product6/1
  Trigonometric Function4/1 -> Product1/2
  Add2/1 -> Mux1/3
  Product5/1 -> Add2/1
  Trigonometric Function2/1 -> Product/3
  Trigonometric Function27/1 -> Product16/2
  Trigonometric Function12/1 -> Product6/2
  Trigonometric Function9/1 -> Product5/2
  Trigonometric Function10/1 -> Product5/3
  Product/1 -> Add1/1
  Reshape1/1 -> Matrix Concatenate/2

== system crazyflie_simulation_paper/G1 ==
  p q r : Inport
  "  2" : Constant  Value=[I_rzz -I_rzz I_rzz -I_rzz; -I_rzz I_rzz -I_rzz I_rzz; 0 0 0 0 ]
  "  3" : Constant  Value=|
      | [-b*k_f  b*k_f  b*k_f  -b*k_f
      | ;  l*k_f  l*k_f -l*k_f  -l*k_f; k_m   -k_m    k_m    -k_m]
  Add : Sum  Inputs=+-
  Constant : Constant  Value=[k_f, k_f, k_f, k_f]
  Constant1 : Constant  Value=I_CF_1_inv
  Demux : Demux  Outputs=3
  Gain : Gain  Gain=[1 0 0]
  Gain1 : Gain  Gain=[0 1 0]
  Gain2 : Gain  Gain=[0 0 0]
  Matrix Concatenate : Concatenate  NumInputs=3  Mode=Multidimensional array
  Matrix Concatenate1 : Concatenate  Mode=Multidimensional array
  Matrix Multiply : Product  Multiplication=Matrix(*)
  Matrix Multiply1 : Product  Multiplication=Matrix(*)
  Reshape{,1..3} (4 alike) : Reshape  OutputDimensionality=Row vector (2-D)
  G1 : Outport
  wires:
  Demux/1 -> Gain/1  "p"
  Gain/1 -> Reshape/1
  Matrix Concatenate/1 -> Matrix Multiply/1
  Demux/2 -> Gain1/1  "q"
  Reshape1/1 -> Matrix Concatenate/2
  Constant/1 -> Reshape3/1
  Reshape2/1 -> Matrix Concatenate/3
  Add/1 -> Matrix Multiply1/2
  Gain2/1 -> Reshape2/1
  "  2"/1 -> Matrix Multiply/2
  Reshape3/1 -> Matrix Concatenate1/2
  Matrix Multiply/1 -> Add/2
  "  3"/1 -> Add/1
  Gain1/1 -> Reshape1/1
  Demux/3 -> Gain2/1  "r"
  Reshape/1 -> Matrix Concatenate/1
  Matrix Concatenate1/1 -> G1/1  "G1"
  p q r/1 -> Demux/1
  Matrix Multiply1/1 -> Matrix Concatenate1/1
  Constant1/1 -> Matrix Multiply1/1

== system crazyflie_simulation_paper/G2 ==
  "  " : Constant  Value=[0 0 0 0; 0 0 0 0; I_rzz -I_rzz I_rzz -I_rzz]
  Constant : Constant  Value=I_CF_1_inv
  Constant1 : Constant  Value=[0, 0, 0, 0]
  Gain1 : Gain  Gain=Ts
  Gain3 : Gain  Gain=-1
  Matrix Concatenate2 : Concatenate  Mode=Multidimensional array
  Matrix Multiply : Product  Multiplication=Matrix(*)
  Reshape4 : Reshape  OutputDimensionality=Row vector (2-D)
  G2 : Outport
  wires:
  Gain3/1 -> Gain1/1
  "  "/1 -> Gain3/1
  Reshape4/1 -> Matrix Concatenate2/2
  Constant1/1 -> Reshape4/1
  Matrix Concatenate2/1 -> G2/1  "G2"
  Gain1/1 -> Matrix Multiply/2
  Constant/1 -> Matrix Multiply/1
  Matrix Multiply/1 -> Matrix Concatenate2/1

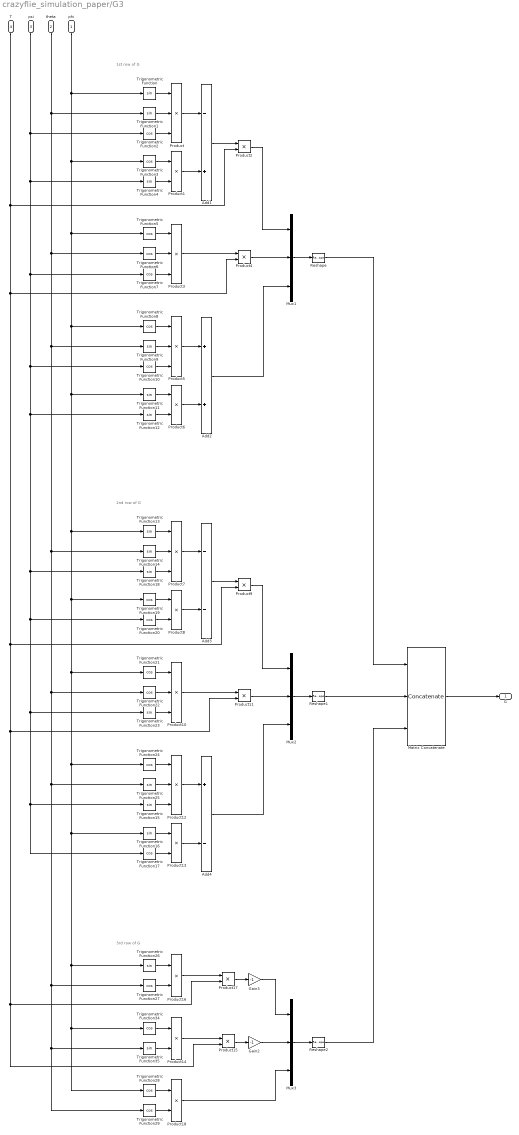
== system crazyflie_simulation_paper/G3 ==
  note: 1st row of G
  note: 2nd row of G
  note: 3rd row of G
  phi : Inport
  theta : Inport  Port=2
  psi : Inport  Port=3
  T : Inport  Port=4
  Add1 : Sum  Inputs=-+
  Add2 : Sum
  Add3 : Sum  Inputs=--
  Add4 : Sum  Inputs=+-
  Gain2 : Gain  Gain=-1
  Gain3 : Gain  Gain=-1
  Matrix Concatenate : Concatenate  NumInputs=3  Mode=Multidimensional array
  Mux1 : Mux  Inputs=3
  Mux2 : Mux  Inputs=3
  Mux3 : Mux  Inputs=3
  Product{,3,5,7,10,12} (6 alike) : Product  Inputs=3
  Product{1..2,4,6,8..9,11,13..18} (13 alike) : Product
  Reshape : Reshape  OutputDimensionality=Row vector (2-D)
  Reshape1 : Reshape  OutputDimensionality=Row vector (2-D)
  Reshape2 : Reshape  OutputDimensionality=Row vector (2-D)
  Trigonometric Function{,1,4,9,11..16,18,23,25..26,35} (15 alike) : Trigonometry
  Trigonometric Function{2..3,5..8,10,17,19..22,24,27..29,34} (17 alike) : Trigonometry  Operator=cos
  G : Outport
  wires:
  T/1 -> Product2/2, Product4/2, Product9/2, Product11/2, Product17/2, Product15/2
  Mux1/1 -> Reshape/1
  theta/1 -> Trigonometric Function1/1, Trigonometric Function6/1, Trigonometric Function9/1, Trigonometric Function14/1, Trigonometric Function22/1, Trigonometric Function25/1, Trigonometric Function27/1, Trigonometric Function35/1, Trigonometric Function29/1
  Trigonometric Function34/1 -> Product14/1
  Reshape/1 -> Matrix Concatenate/1
  psi/1 -> Trigonometric Function2/1, Trigonometric Function4/1, Trigonometric Function7/1, Trigonometric Function10/1, Trigonometric Function12/1, Trigonometric Function18/1, Trigonometric Function20/1, Trigonometric Function23/1, Trigonometric Function15/1, Trigonometric Function17/1
  Trigonometric Function25/1 -> Product12/2
  Trigonometric Function26/1 -> Product16/1
  Add1/1 -> Product2/1
  phi/1 -> Trigonometric Function3/1, Trigonometric Function8/1, Trigonometric Function13/1, Trigonometric Function19/1, Trigonometric Function21/1, Trigonometric Function24/1, Trigonometric Function26/1, Trigonometric Function34/1, Trigonometric Function28/1, Trigonometric Function16/1, Trigonometric Function11/1, Trigonometric Function5/1, Trigonometric Function/1
  Trigonometric Function15/1 -> Product12/3
  Trigonometric Function24/1 -> Product12/1
  Trigonometric Function20/1 -> Product8/2
  Product18/1 -> Mux3/3
  Product4/1 -> Mux1/2
  Mux3/1 -> Reshape2/1
  Product7/1 -> Add3/1
  Trigonometric Function6/1 -> Product3/2
  Matrix Concatenate/1 -> G/1
  Trigonometric Function7/1 -> Product3/3
  Trigonometric Function3/1 -> Product1/1
  Trigonometric Function29/1 -> Product18/2
  Trigonometric Function5/1 -> Product3/1
  Product1/1 -> Add1/2
  Trigonometric Function8/1 -> Product5/1
  Product6/1 -> Add2/2
  Product15/1 -> Gain2/1
  Mux2/1 -> Reshape1/1
  Product17/1 -> Gain3/1
  Gain2/1 -> Mux3/2
  Trigonometric Function17/1 -> Product13/2
  Product12/1 -> Add4/1
  Trigonometric Function19/1 -> Product8/1
  Product3/1 -> Product4/1
  Product9/1 -> Mux2/1
  Product16/1 -> Product17/1
  Add4/1 -> Mux2/3
  Trigonometric Function16/1 -> Product13/1
  Product8/1 -> Add3/2
  Trigonometric Function13/1 -> Product7/1
  Trigonometric Function28/1 -> Product18/1
  Gain3/1 -> Mux3/1
  Add3/1 -> Product9/1
  Trigonometric Function35/1 -> Product14/2
  Trigonometric Function18/1 -> Product7/3
  Product14/1 -> Product15/1
  Trigonometric Function/1 -> Product/1
  Product11/1 -> Mux2/2
  Product13/1 -> Add4/2
  Trigonometric Function21/1 -> Product10/1
  Product10/1 -> Product11/1
  Trigonometric Function22/1 -> Product10/2
  Trigonometric Function23/1 -> Product10/3
  Trigonometric Function14/1 -> Product7/2
  Reshape2/1 -> Matrix Concatenate/3
  Trigonometric Function1/1 -> Product/2
  Product2/1 -> Mux1/1
  Trigonometric Function11/1 -> Product6/1
  Trigonometric Function4/1 -> Product1/2
  Add2/1 -> Mux1/3
  Product5/1 -> Add2/1
  Trigonometric Function2/1 -> Product/3
  Trigonometric Function27/1 -> Product16/2
  Trigonometric Function12/1 -> Product6/2
  Trigonometric Function9/1 -> Product5/2
  Trigonometric Function10/1 -> Product5/3
  Product/1 -> Add1/1
  Reshape1/1 -> Matrix Concatenate/2

== system crazyflie_simulation_paper/G4 ==
  p q r : Inport
  "  2" : Constant  Value=[I_rzz -I_rzz I_rzz -I_rzz; -I_rzz I_rzz -I_rzz I_rzz; 0 0 0 0 ]
  "  3" : Constant  Value=|
      | [-b*k_f  b*k_f  b*k_f  -b*k_f
      | ;  l*k_f  l*k_f -l*k_f  -l*k_f; k_m   -k_m    k_m    -k_m]
  Add : Sum  Inputs=+-
  Constant : Constant  Value=[k_f, k_f, k_f, k_f]
  Constant1 : Constant  Value=I_CF_1_inv
  Demux : Demux  Outputs=3
  Gain : Gain  Gain=[1 0 0]
  Gain1 : Gain  Gain=[0 1 0]
  Gain2 : Gain  Gain=[0 0 0]
  Matrix Concatenate : Concatenate  NumInputs=3  Mode=Multidimensional array
  Matrix Concatenate1 : Concatenate  Mode=Multidimensional array
  Matrix Multiply : Product  Multiplication=Matrix(*)
  Matrix Multiply1 : Product  Multiplication=Matrix(*)
  Reshape{,1..3} (4 alike) : Reshape  OutputDimensionality=Row vector (2-D)
  G1 : Outport
  wires:
  Demux/1 -> Gain/1  "p"
  Gain/1 -> Reshape/1
  Matrix Concatenate/1 -> Matrix Multiply/1
  Demux/2 -> Gain1/1  "q"
  Reshape1/1 -> Matrix Concatenate/2
  Constant/1 -> Reshape3/1
  Reshape2/1 -> Matrix Concatenate/3
  Add/1 -> Matrix Multiply1/2
  Gain2/1 -> Reshape2/1
  "  2"/1 -> Matrix Multiply/2
  Reshape3/1 -> Matrix Concatenate1/2
  Matrix Multiply/1 -> Add/2
  "  3"/1 -> Add/1
  Gain1/1 -> Reshape1/1
  Demux/3 -> Gain2/1  "r"
  Reshape/1 -> Matrix Concatenate/1
  Matrix Concatenate1/1 -> G1/1  "G1"
  p q r/1 -> Demux/1
  Matrix Multiply1/1 -> Matrix Concatenate1/1
  Constant1/1 -> Matrix Multiply1/1

== system crazyflie_simulation_paper/G5 ==
  "  " : Constant  Value=[0 0 0 0; 0 0 0 0; I_rzz -I_rzz I_rzz -I_rzz]
  Constant : Constant  Value=I_CF_1_inv
  Constant1 : Constant  Value=[0, 0, 0, 0]
  Gain1 : Gain  Gain=Ts
  Gain3 : Gain  Gain=-1
  Matrix Concatenate2 : Concatenate  Mode=Multidimensional array
  Matrix Multiply : Product  Multiplication=Matrix(*)
  Reshape4 : Reshape  OutputDimensionality=Row vector (2-D)
  G2 : Outport
  wires:
  Gain3/1 -> Gain1/1
  "  "/1 -> Gain3/1
  Reshape4/1 -> Matrix Concatenate2/2
  Constant1/1 -> Reshape4/1
  Matrix Concatenate2/1 -> G2/1  "G2"
  Gain1/1 -> Matrix Multiply/2
  Constant/1 -> Matrix Multiply/1
  Matrix Multiply/1 -> Matrix Concatenate2/1

== system crazyflie_simulation_paper/Signal Builder1 ==
  Demux : Demux  Tag=STV Demux  Outputs=3
  FromWs : FromWorkspace  Tag=STV FromWs  VariableName=tuvar  SampleTime=0
      SigBuilderData=|
      | common.afterFinalStr = 'Extrapolate'
      | common.sampleTime = 0
      | dataSet.timeRange = [0 50]
      | dataSet.name = 'Group 1'
      | sbobj.Groups.Name = 'Group 1'
      | sbobj.Groups.Signals(1).Name = 'Signal 1'
      | sbobj.Groups.Signals(1).XData = [0 2 2 10 10 20 20 27 27 30 40 40 50]
      | sbobj.Groups.Signals(1).YData = [0 0 3.01 3.01 5 5 1.98 1.98 3.5 3.5 3.5 0 0]
      | sbobj.Groups.Signals(2).Name = 'Signal 2'
      | sbobj.Groups.Signals(2).XData = [0 5 7.6 7.6 25 25 27 35 35 45 45 50]
      | sbobj.Groups.Signals(2).YData = [0 0 0 3 3 0.4 0.4 0.4 3.49 3.49 0 0]
      | sbobj.Groups.Signals(3).Name = 'Signal 3'
      | sbobj.Groups.Signals(3).XData = [0 1 1 23.5 23.5 40 40 50]
      | sbobj.Groups.Signals(3).YData = [0 0 7 7 5 5 0 0]
      | sbobj.Groups.TimeRange = [0 50]
  Signal 1 : Outport  Tag=STV Outport
  Signal 2 : Outport  Tag=STV Outport  Port=2
  Signal 3 : Outport  Tag=STV Outport  Port=3
  wires:
  Demux/3 -> Signal 3/1
  Demux/2 -> Signal 2/1
  Demux/1 -> Signal 1/1
  FromWs/1 -> Demux/1

== system crazyflie_simulation_paper/Signal Builder2 ==
  Demux : Demux  Tag=STV Demux  Outputs=3
  FromWs : FromWorkspace  Tag=STV FromWs  VariableName=tuvar  SampleTime=0
      SigBuilderData=|
      | common.afterFinalStr = 'Extrapolate'
      | common.sampleTime = 0
      | dataSet.timeRange = [0 50]
      | dataSet.name = 'Group 1'
      | sbobj.Groups.Name = 'Group 1'
      | sbobj.Groups.Signals(1).Name = 'Signal 1'
      | sbobj.Groups.Signals(1).XData = [0 2 2 10 10 20 20 27 27 30 40 40 50]
      | sbobj.Groups.Signals(1).YData = [0 0 3.01 3.01 5 5 1.98 1.98 3.5 3.5 3.5 0 0]
      | sbobj.Groups.Signals(2).Name = 'Signal 2'
      | sbobj.Groups.Signals(2).XData = [0 5 7.6 7.6 25 25 27 35 35 45 45 50]
      | sbobj.Groups.Signals(2).YData = [0 0 0 3 3 0.4 0.4 0.4 3.49 3.49 0 0]
      | sbobj.Groups.Signals(3).Name = 'Signal 3'
      | sbobj.Groups.Signals(3).XData = [0 1 1 23.5 23.5 40 40 50]
      | sbobj.Groups.Signals(3).YData = [0 0 7 7 5 5 0 0]
      | sbobj.Groups.TimeRange = [0 50]
  Signal 1 : Outport  Tag=STV Outport
  Signal 2 : Outport  Tag=STV Outport  Port=2
  Signal 3 : Outport  Tag=STV Outport  Port=3
  wires:
  FromWs/1 -> Demux/1
  Demux/1 -> Signal 1/1
  Demux/2 -> Signal 2/1
  Demux/3 -> Signal 3/1

== system crazyflie_simulation_paper/Signal Builder3 ==
  Demux : Demux  Tag=STV Demux  Outputs=3
  FromWs : FromWorkspace  Tag=STV FromWs  VariableName=tuvar  SampleTime=0
      SigBuilderData=|
      | common.afterFinalStr = 'Extrapolate'
      | common.sampleTime = 0
      | dataSet.timeRange = [0 50]
      | dataSet.name = 'Group 1'
      | sbobj.Groups.Name = 'Group 1'
      | sbobj.Groups.Signals(1).Name = 'Signal 1'
      | sbobj.Groups.Signals(1).XData = [0 2 2 10 10 20 20 27 27 30 40 40 50]
      | sbobj.Groups.Signals(1).YData = [0 0 3.01 3.01 5 5 1.98 1.98 3.5 3.5 3.5 0 0]
      | sbobj.Groups.Signals(2).Name = 'Signal 2'
      | sbobj.Groups.Signals(2).XData = [0 5 7.6 7.6 25 25 27 35 35 45 45 50]
      | sbobj.Groups.Signals(2).YData = [0 0 0 3 3 0.4 0.4 0.4 3.49 3.49 0 0]
      | sbobj.Groups.Signals(3).Name = 'Signal 3'
      | sbobj.Groups.Signals(3).XData = [0 1 1 23.5 23.5 40 40 50]
      | sbobj.Groups.Signals(3).YData = [0 0 7 7 5 5 0 0]
      | sbobj.Groups.TimeRange = [0 50]
  Signal 1 : Outport  Tag=STV Outport
  Signal 2 : Outport  Tag=STV Outport  Port=2
  Signal 3 : Outport  Tag=STV Outport  Port=3
  wires:
  FromWs/1 -> Demux/1
  Demux/1 -> Signal 1/1
  Demux/2 -> Signal 2/1
  Demux/3 -> Signal 3/1

== system crazyflie_simulation_paper/Crazyflie Quadrotor Dynamics/Aerodynamic Force ==
  V_B : Inport
  Demux : Demux  Outputs=3
  Gain : Gain  Gain=-kx
  Gain1 : Gain  Gain=-ky
  Gain2 : Gain  Gain=-kz
  Mux1 : Mux  Inputs=3
  Reshape : Reshape  OutputDimensionality=Column vector (2-D)
  FA_B : Outport
  wires:
  Reshape/1 -> FA_B/1  "FA_B"
  Demux/1 -> Gain/1  "v_B"
  Demux/3 -> Gain2/1  "w_B"
  V_B/1 -> Demux/1
  Demux/2 -> Gain1/1  "u_B"
  Gain/1 -> Mux1/1
  Gain1/1 -> Mux1/2
  Mux1/1 -> Reshape/1
  Gain2/1 -> Mux1/3

== system crazyflie_simulation_paper/Crazyflie Quadrotor Dynamics/Cross Product Custom ==
  A : Inport
  B : Inport  Port=2
  A1 : InportShadow
  B1 : InportShadow  Port=2
  Subsystem : sharedutil/3x3 Cross Product/Subsystem  SystemSampleTime=-1
      settings: SourceProductName=Aerospace Blockset  SourceProductBaseCode=AE
  Subsystem1 : sharedutil/3x3 Cross Product/Subsystem1  SystemSampleTime=-1
      settings: SourceProductName=Aerospace Blockset  SourceProductBaseCode=AE
  Sum3 : Sum  Inputs=+|-  SaturateOnIntegerOverflow=on  InputSameDT=on  OutDataTypeStr=Inherit: Same as first input
  C : Outport
  wires:
  Subsystem/1 -> Sum3/1
  B1/1 -> Subsystem1/2
  Sum3/1 -> C/1
  B/1 -> Subsystem/2
  Subsystem1/1 -> Sum3/2
  A/1 -> Subsystem/1
  A1/1 -> Subsystem1/1

== system crazyflie_simulation_paper/Crazyflie Quadrotor Dynamics/Gravitational Force  ==
  Product : Product
  Reshape : Reshape  OutputDimensionality=Column vector (2-D)
  g_acc : Constant  Value=[0; 0; g]
  m_CF : Constant  Value=m_CF
  FG_O : Outport
  wires:
  Reshape/1 -> FG_O/1  "FG_O"
  Product/1 -> Reshape/1
  g_acc/1 -> Product/1
  m_CF/1 -> Product/2

== system crazyflie_simulation_paper/Crazyflie Quadrotor Dynamics/Propulsive Force ==
  omegaR : Inport
  Constant : Constant  Value=0
  Demux1 : Demux
  Gain4 : Gain  Gain=-k_f
  Matrix Sum2 : Sum  Inputs=++++
  Mux : Mux  Inputs=3
  Reshape : Reshape  OutputDimensionality=Column vector (2-D)
  FP_B : Outport
  wires:
  Constant/1 -> Mux/1, Mux/2
  Reshape/1 -> FP_B/1  "FP_B"
  Demux1/3 -> Matrix Sum2/3  "omegaR_3"
  Demux1/1 -> Matrix Sum2/1  "omegaR_1"
  Demux1/4 -> Matrix Sum2/4  "omegaR_4"
  Mux/1 -> Reshape/1
  Matrix Sum2/1 -> Gain4/1
  omegaR/1 -> Demux1/1
  Demux1/2 -> Matrix Sum2/2  "omegaR_2"
  Gain4/1 -> Mux/3
